simulink subsystem "Controls"  (R2024b)
settings: Solver=VariableStepAuto  StartTime=0.0  StopTime=10.0  RelTol=1e-3
undefined symbols (not defined in the file): D1, DiscIntNeverNeededParam, lag, Tctrl, test_alpha, Ts, Yg
libraries: powerlib_extras x74, simulink x10
(part 1 of 7)
settings Model: ModifiedByFormat=Kyle  Creator=Kyle  LastModifiedBy=Kyle

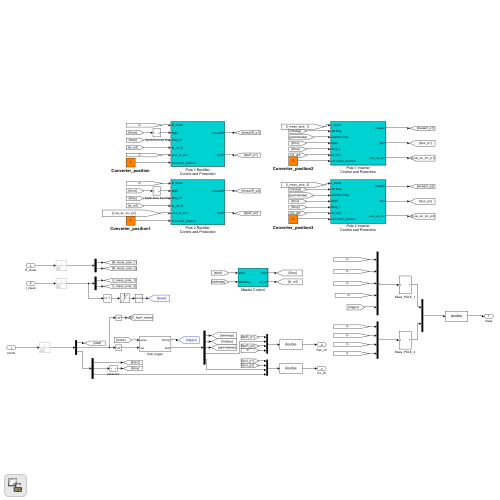
[thumbnail: Simulink's stored preview of the top-level diagram]
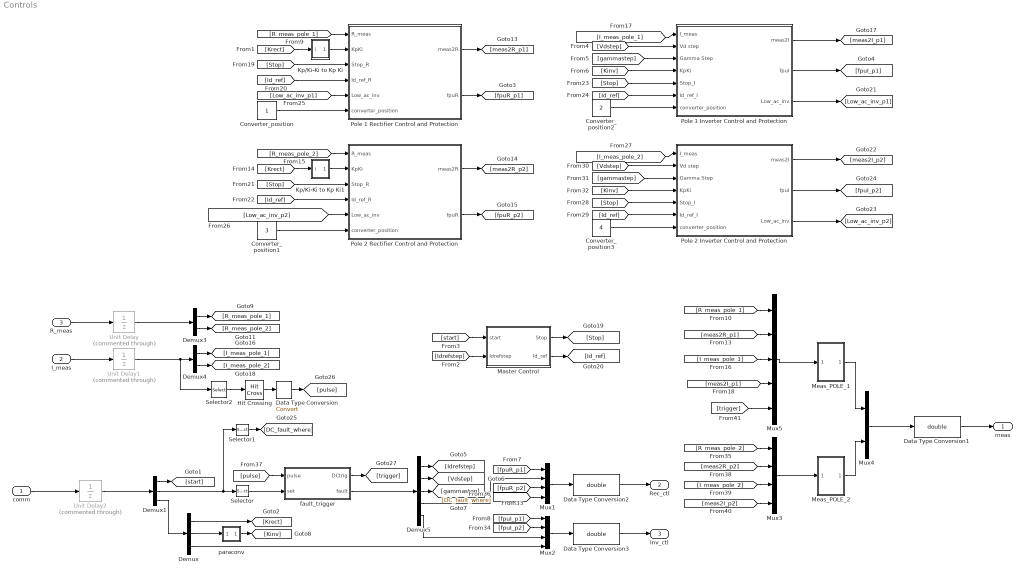
== system Controls ==
  comm : Inport
  I_meas : Inport  Port=2
  R_meas : Inport  Port=3
  Converter_position : Constant
  Converter_position1 : Constant  Value=3
  Converter_position2 : Constant  Value=2
  Converter_position3 : Constant  Value=4
  Data Type Conversion : DataTypeConversion  SaturateOnIntegerOverflow=off  RndMeth=Floor
  Data Type Conversion1 : DataTypeConversion  OutDataTypeStr=double  SaturateOnIntegerOverflow=off  RndMeth=Floor  LockScale=on
  Data Type Conversion2 : DataTypeConversion  OutDataTypeStr=double  SaturateOnIntegerOverflow=off  RndMeth=Floor
  Data Type Conversion3 : DataTypeConversion  OutDataTypeStr=double  SaturateOnIntegerOverflow=off  RndMeth=Floor  LockScale=on
  Demux : Demux  Outputs=[2 6 5]
  Demux1 : Demux  Outputs=[1 16 13]
  Demux3 : Demux  Outputs=[14 14]
  Demux4 : Demux  Outputs=[24 24]
  Demux5 : Demux  Outputs=[1 1 1 2 3]
  Hit Crossing : HitCross  HitCrossingDirection=rising
  Kp/Ki-Ki to Kp Ki : Subsystem
  Kp/Ki-Ki to Kp Ki1 : Subsystem
  Master Control : Subsystem
  Meas_POLE_1 : Subsystem
  Meas_POLE_2 : Subsystem
  Mux1 : Mux  Inputs=[6 2 6 1]
  Mux2 : Mux  Inputs=[6 6 3 5]
  Mux3 : Mux  Inputs=[14 6 24 12 ]
  Mux4 : Mux  Inputs=[57 56]
  Mux5 : Mux  Inputs=[14 6 24 12 1]
  Pole 1 Inverter Control and Protection : Subsystem
  Pole 1 Rectifier Control and Protection : Subsystem
  Pole 2 Inverter Control and Protection : Subsystem
  Pole 2 Rectifier Control and Protection : Subsystem
  Selector : Selector  IndexOptions=Index vector (dialog)  Indices=[1:4, 6:16]  OutputSizes=1
  Selector1 : Selector  IndexOptions=Index vector (dialog)  Indices=[5]  OutputSizes=1
  Selector2 : Selector  IndexOptions=Index vector (dialog)  Indices=1  OutputSizes=1
  Unit Delay : UnitDelay  Commented=through  SampleTime=Ts  HasFrameUpgradeWarning=on
  Unit Delay1 : UnitDelay  Commented=through  SampleTime=Ts  HasFrameUpgradeWarning=on
  Unit Delay2 : UnitDelay  Commented=through  SampleTime=Ts  HasFrameUpgradeWarning=on
  fault_trigger : Subsystem
  paraconv : Subsystem
  meas : Outport
  Rec_ctl : Outport  Port=2
  Inv_ctl : Outport  Port=3
  wires:
  Demux1/1 -> [start]
  [start] -> Master Control/1(start)
  [Idrefstep] -> Master Control/2(Idrefstep)
  [Vdstep] -> Pole 1 Inverter Control and Protection/2(Vd step)
  [gammastep] -> Pole 1 Inverter Control and Protection/3(Gamma Step)
  Pole 1 Inverter Control and Protection/2(fpuI) -> [fpuI_p1]
  Pole 1 Rectifier Control and Protection/2(fpuR) -> [fpuR_p1]
  [Kinv] -> Pole 1 Inverter Control and Protection/4(KpKi)
  Kp/Ki-Ki to Kp Ki/1(o) -> Pole 1 Rectifier Control and Protection/2(KpKi)
  Demux/3 -> Mux2/4
  Demux1/3 -> Demux/1
  [Krect] -> Kp/Ki-Ki to Kp Ki/1(i)
  Demux/1 -> [Krect]
  Demux/2 -> paraconv/1(In1)
  comm/1 -> Unit Delay2/1
  Demux5/1 -> [Idrefstep]
  Demux5/2 -> [Vdstep]
  Demux5/3 -> [gammastep]
  Demux1/2 -> Selector1/1, Selector/1
  paraconv/1(Out1) -> [Kinv]
  [fpuR_p1] -> Mux1/1
  [fpuI_p1] -> Mux2/1
  Demux5/5 -> Mux2/3
  R_meas/1 -> Unit Delay/1
  I_meas/1 -> Unit Delay1/1
  Mux5/1 -> Meas_POLE_1/1(In1)
  Demux3/1 -> [R_meas_pole_1]
  Demux3/2 -> [R_meas_pole_2]
  [R_meas_pole_1] -> Mux5/1
  [R_meas_pole_1] -> Pole 1 Rectifier Control and Protection/1(R_meas)
  Pole 1 Rectifier Control and Protection/1(meas2R) -> [meas2R_p1]
  [meas2R_p1] -> Mux5/2
  Converter_position/1 -> Pole 1 Rectifier Control and Protection/6(converter_position)
  Pole 2 Rectifier Control and Protection/2(fpuR) -> [fpuR_p2]
  Kp/Ki-Ki to Kp Ki1/1(o) -> Pole 2 Rectifier Control and Protection/2(KpKi)
  [Krect] -> Kp/Ki-Ki to Kp Ki1/1(i)
  [R_meas_pole_2] -> Pole 2 Rectifier Control and Protection/1(R_meas)
  Pole 2 Rectifier Control and Protection/1(meas2R) -> [meas2R_p2]
  Converter_position1/1 -> Pole 2 Rectifier Control and Protection/6(converter_position)
  Demux4/1 -> [I_meas_pole_1]
  [I_meas_pole_1] -> Mux5/3
  [I_meas_pole_1] -> Pole 1 Inverter Control and Protection/1(I_meas)
  Pole 1 Inverter Control and Protection/1(meas2I) -> [meas2I_p1]
  [meas2I_p1] -> Mux5/4
  Demux4/2 -> [I_meas_pole_2]
  Converter_position2/1 -> Pole 1 Inverter Control and Protection/7(converter_position)
  Master Control/2(Id_ref) -> [Id_ref]
  Master Control/1(Stop) -> [Stop]
  Pole 1 Inverter Control and Protection/3(Low_ac_inv) -> [Low_ac_inv_p1]
  [Low_ac_inv_p1] -> Pole 1 Rectifier Control and Protection/5(Low_ac_inv)
  [Low_ac_inv_p2] -> Pole 2 Rectifier Control and Protection/5(Low_ac_inv)
  [Vdstep] -> Pole 2 Inverter Control and Protection/2(Vd step)
  [gammastep] -> Pole 2 Inverter Control and Protection/3(Gamma Step)
  Pole 2 Inverter Control and Protection/2(fpuI) -> [fpuI_p2]
  [Kinv] -> Pole 2 Inverter Control and Protection/4(KpKi)
  [I_meas_pole_2] -> Pole 2 Inverter Control and Protection/1(I_meas)
  Pole 2 Inverter Control and Protection/1(meas2I) -> [meas2I_p2]
  Converter_position3/1 -> Pole 2 Inverter Control and Protection/7(converter_position)
  Pole 2 Inverter Control and Protection/3(Low_ac_inv) -> [Low_ac_inv_p2]
  [fpuI_p2] -> Mux2/2
  Mux3/1 -> Meas_POLE_2/1(In1)
  [R_meas_pole_2] -> Mux3/1
  [meas2R_p2] -> Mux3/2
  [I_meas_pole_2] -> Mux3/3
  [meas2I_p2] -> Mux3/4
  Meas_POLE_1/1(Out1) -> Mux4/1
  Meas_POLE_2/1(Out1) -> Mux4/2
  Mux4/1 -> Data Type Conversion1/1
  [Stop] -> Pole 2 Rectifier Control and Protection/3(Stop_R)
  [Id_ref] -> Pole 2 Rectifier Control and Protection/4(Id_ref_R)
  [Id_ref] -> Pole 1 Inverter Control and Protection/6(Id_ref_I)
  [Stop] -> Pole 1 Inverter Control and Protection/5(Stop_I)
  [Stop] -> Pole 2 Inverter Control and Protection/5(Stop_I)
  [Id_ref] -> Pole 2 Inverter Control and Protection/6(Id_ref_I)
  [fpuR_p2] -> Mux1/3
  Demux5/4 -> Mux1/2
  [Stop] -> Pole 1 Rectifier Control and Protection/3(Stop_R)
  [Id_ref] -> Pole 1 Rectifier Control and Protection/4(Id_ref_R)
  Selector/1 -> fault_trigger/2(set)
  [DC_fault_where] -> Mux1/4
  Selector1/1 -> [DC_fault_where]
  fault_trigger/2(fault) -> Demux5/1
  fault_trigger/1(DCtrig) -> [trigger]
  [pulse] -> fault_trigger/1(pulse)
  [trigger] -> Mux5/5
  Hit Crossing/1 -> Data Type Conversion/1
  Data Type Conversion/1 -> [pulse]
  Selector2/1 -> Hit Crossing/1
  Unit Delay/1 -> Demux3/1
  Unit Delay1/1 -> Demux4/1, Selector2/1
  Unit Delay2/1 -> Demux1/1
  Data Type Conversion1/1 -> meas/1
  Mux2/1 -> Data Type Conversion3/1
  Mux1/1 -> Data Type Conversion2/1
  Data Type Conversion2/1 -> Rec_ctl/1
  Data Type Conversion3/1 -> Inv_ctl/1

== system Controls/Kp//Ki-Ki to Kp Ki ==
  i : Inport
  Mux3 : Mux  Inputs=2
  Product11 : Product  Inputs=1  RndMeth=Zero
  Selector12 : Selector  InputPortWidth=2  IndexOptions=Index vector (dialog)  Indices=2  OutputSizes=1
  o : Outport
  wires:
  Mux3/1 -> o/1
  Selector12/1 -> Mux3/2
  Product11/1 -> Mux3/1
  i/1 -> Product11/1, Selector12/1

== system Controls/Kp//Ki-Ki to Kp Ki1 ==
  i : Inport
  Mux3 : Mux  Inputs=2
  Product11 : Product  Inputs=1  RndMeth=Zero
  Selector12 : Selector  InputPortWidth=2  IndexOptions=Index vector (dialog)  Indices=2  OutputSizes=1
  o : Outport
  wires:
  Mux3/1 -> o/1
  Selector12/1 -> Mux3/2
  Product11/1 -> Mux3/1
  i/1 -> Product11/1, Selector12/1

== system Controls/Master Control ==
  note: Master Control
  start : Inport
  Idrefstep : Inport  Port=2
  Constant : Constant  Value=0
  Discrete Monostable1 : powerlib_extras/Discrete  Control Blocks/Discrete Monostable  EdgeDetect=Rising  t_mono=0.1  ic=0  Ts=Tctrl
  Informations : Subsystem
      mask Display: disp('?')
  Product : Product  RndMeth=Zero
  Start/Stop : Subsystem  mask(Start/Stop  & Ramping){Min_ref=0.1, X_start=[0.3333, 0.02], X_up=[5.0, 0.4, 1.0], X_down=[-5.0,  1.4], T_stop=1.6, dt=Tctrl}
      mask prompts: Min_ref "Minimum Steady-State Current Reference (pu):"; X_start "{Start Ramp}: [Rate (pu/s), Time (s)]"; X_up "{Up Ramp}: [Rate (pu/s), Time (s), Final Value (pu)]"; X_down "{Down Ramp}: [Rate (-pu/s), Time (s)]"; T_stop "Stop Time (s):"; dt "Sample Time (s):"
      mask help:
      | At start-up, both converters are deblocked and ramped up to the minimum current (Minimum Steady-State Current Reference) with an adjustable rate (Start Ramp Rate) and application time (Start Ramp Time).
      |
      | After the system stabilisation the current is ramped up to its final value (Up Ramp Final Value) with an adjustable rate (Up Ramp Rate) and execution time (Up Ramp Time).
      |
      | Before stopping the converters (at Stop Time) the current is ramped down to the minimum current  with an adjustable rate (Down Ramp Rate) and execution time  (Down Ramp Time).
      |
      | At Stop Time the reference is ramped down to zero with the same rate used for the Start Ramp.
      mask init:
      | T_up = X_up(2); F_up = X_up(3); up_slope = X_up(1);
      | T_up_final =  T_up + (F_up - Min_ref)/up_slope;
      | 
      | T_down = X_down(2); F_down = Min_ref; down_slope = X_down(1);
      | T_down_final =   T_down + (F_down-F_up)/down_slope;
      | 
      | SS_ramp = X_start(1); T_start = X_start(2);
      | 
      | T_ramp  = [0, T_up, T_up_final,  T_down,  T_down_final, 9999]';
      | U_ramp = [0, 0, F_up-Min_ref,  F_up-Min_ref,  F_down- Min_ref,  F_down - Min_ref]';
      mask Display: disp('Start/Stop\n & Ramping')
  Step : Step  Time=0.1  SampleTime=Tctrl
  Sum : Sum  SaturateOnIntegerOverflow=on
  Sum1 : Sum  SaturateOnIntegerOverflow=on
  g : Gain  Gain=-0.2  SaturateOnIntegerOverflow=on  OutDataTypeStr=Inherit: Same as input  ParamDataTypeStr=Inherit: Same as input
  Stop : Outport
  Id_ref : Outport  Port=2
  wires:
  Start/Stop/2("Stop ") -> Stop/1
  Step/1 -> Product/1
  Product/1 -> Start/Stop/1(start)
  start/1 -> Product/2
  Idrefstep/1 -> Discrete Monostable1/1
  g/1 -> Sum1/2
  Discrete Monostable1/1 -> g/1
  Start/Stop/1(Id_ref_ramp) -> Sum/1
  Sum/1 -> Id_ref/1
  Sum1/1 -> Sum/2
  Constant/1 -> Sum1/1

== system Controls/Meas_POLE_1 ==
  In1 : Inport
  Demux1 : Demux  Outputs="[14 6 24 12  1]"
      settings: DisplayOption=none
  Demux3 : Demux  Outputs=12
      settings: DisplayOption=none
  Demux4 : Demux  Outputs=14
      settings: DisplayOption=none
  Demux5 : Demux  Outputs=6
      settings: DisplayOption=none
  Demux6 : Demux  Outputs=24
      settings: DisplayOption=none
  Mux1 : Mux  Inputs="[14 6 24 12  1]"
  Mux3 : Mux  Inputs=12
  Mux4 : Mux  Inputs=14
  Mux5 : Mux  Inputs=24
  Mux6 : Mux  Inputs=6
  Out1 : Outport
  wires:
  Demux6/24 -> Mux5/24  "Iac fault (A)"
  Demux4/14 -> Mux4/14  "Idc fault (A)"
  Demux1/2 -> Demux5/1
  Mux6/1 -> Mux1/2
  Demux5/1 -> Mux6/1  "Vdc_Rect (pu/500kV)"
  Demux5/2 -> Mux6/2  "Id_ref_limit_Rect"
  Demux5/3 -> Mux6/3  "alpha Rect (degree)"
  Demux5/4 -> Mux6/4  "Mode"
  Demux5/5 -> Mux6/5  "Low AC voltage Rect"
  Demux5/6 -> Mux6/6  "Forced alpha Rect"
  Demux1/1 -> Demux4/1
  Demux4/13 -> Mux4/13  "Vdc_neutral (pu/500kV)"
  Demux4/12 -> Mux4/12  "Ithy1 D Rect (pu/1kA)"
  Demux4/11 -> Mux4/11  "Vthy1 D Rect (pu/500kV)"
  Demux4/10 -> Mux4/10  "Ithy1 Y Rect (pu/1kA)"
  Demux4/9 -> Mux4/9  "Vthy1 Y Rect (pu/500kV)"
  Demux4/8 -> Mux4/8  "Id Rect (pu/1kA)"
  Demux4/7 -> Mux4/7  "Vdc Rect (pu/500kV)"
  Mux4/1 -> Mux1/1
  Demux4/6 -> Mux4/6  "Ic Rect (pu/817A)"
  Demux4/5 -> Mux4/5  "Ib Rect (pu/817A)"
  Demux4/4 -> Mux4/4  "Ia Rect (pu/817A)"
  Demux4/3 -> Mux4/3  "Vc_Rect (pu/500kVLL)"
  Demux4/2 -> Mux4/2  "Vb_Rect (pu/500kVLL)"
  Demux4/1 -> Mux4/1  "Va_Rect (pu/500kVLL)"
  Mux3/1 -> Mux1/4
  Demux1/4 -> Demux3/1
  Demux3/12 -> Mux3/12  "Gamma mean"
  Demux3/11 -> Mux3/11  "Vsw1 Inv(pu)"
  Demux3/10 -> Mux3/10  "Isw1 Inv (pu)"
  Demux3/9 -> Mux3/9  "Alpha  min Inv"
  Demux3/8 -> Mux3/8  "Low AC voltage Inv"
  Demux3/7 -> Mux3/7  "Gamma Ref Inv"
  Demux3/6 -> Mux3/6  "Gamma min Inv"
  Demux3/5 -> Mux3/5  "Mode"
  Demux3/4 -> Mux3/4  "alpha Inv (degree)"
  Demux3/3 -> Mux3/3  "Id limite (pu)"
  Demux3/2 -> Mux3/2  "Vd Ref Inv (pu)"
  Demux3/1 -> Mux3/1  "Vdc_Inv (pu/500kV)"
  Demux1/5 -> Mux1/5  "trigger sig"
  In1/1 -> Demux1/1
  Mux1/1 -> Out1/1
  Demux6/23 -> Mux5/23  "Vdc_neutral (pu/500kV)"
  Demux6/22 -> Mux5/22  "V thy 1D (pu/500kV)"
  Demux6/21 -> Mux5/21  "Vthy1Y(pu/500kV)"
  Demux6/20 -> Mux5/20  "I thy 6 D (pu/1kA)"
  Demux6/19 -> Mux5/19  "I thy 5 D (pu/1kA)"
  Demux6/18 -> Mux5/18  "I thy 4 D (pu/1kA)"
  Demux6/17 -> Mux5/17  "I thy 3 D (pu/1kA)"
  Demux6/16 -> Mux5/16  "I thy 2 D (pu/1kA)"
  Demux6/15 -> Mux5/15  "I thy 1 D (pu/1kA)"
  Demux6/14 -> Mux5/14  "I thy 6 Y (pu/1kA)"
  Demux6/1 -> Mux5/1  "Va_Inv (pu/345kVLL)"
  Demux6/2 -> Mux5/2  "Vb_Inv (pu/345kVLL)"
  Demux6/3 -> Mux5/3  "Vc_Inv (pu/345kVLL)"
  Demux6/4 -> Mux5/4  "Ia_Inv (pu/290A)"
  Demux6/5 -> Mux5/5  "Ib_Inv (pu/290A)"
  Demux6/6 -> Mux5/6  "Ic_Inv (pu/290A)"
  Demux1/3 -> Demux6/1
  Mux5/1 -> Mux1/3
  Demux6/7 -> Mux5/7  "Vdc Inv (pu/500kV)"
  Demux6/8 -> Mux5/8  "Idc Inv (pu/1kA)"
  Demux6/9 -> Mux5/9  "I thy 1 Y (pu/1kA)"
  Demux6/10 -> Mux5/10  "I thy 2 Y (pu/1kA)"
  Demux6/11 -> Mux5/11  "I thy 3 Y (pu/1kA)"
  Demux6/12 -> Mux5/12  "I thy 4 Y (pu/1kA)"
  Demux6/13 -> Mux5/13  "I thy 5 Y (pu/1kA)"

== system Controls/Meas_POLE_2 ==
  In1 : Inport
  Demux1 : Demux  Outputs=[14 6 24 12]
      settings: DisplayOption=none
  Demux3 : Demux  Outputs=12
      settings: DisplayOption=none
  Demux4 : Demux  Outputs=14
      settings: DisplayOption=none
  Demux5 : Demux  Outputs=6
      settings: DisplayOption=none
  Demux6 : Demux  Outputs=24
      settings: DisplayOption=none
  Gain{,1..4} (5 alike) : Gain  Gain=-1
  Mux1 : Mux  Inputs=[14 6 24 12 ]
  Mux3 : Mux  Inputs=12
  Mux4 : Mux  Inputs=14
  Mux5 : Mux  Inputs=24
  Mux6 : Mux  Inputs=6
  Out1 : Outport
  wires:
  Gain4/1 -> Mux3/3  "Id limite (pu)"
  Gain3/1 -> Mux3/2  "Vd Ref Inv (pu)"
  Gain2/1 -> Mux3/1  "Vdc_Inv (pu/500kV)"
  Gain1/1 -> Mux6/2  "Id_ref_limit_Rect"
  Gain/1 -> Mux6/1  "Vdc_Rect (pu/500kV)"
  Demux6/24 -> Mux5/24  "Iac fault (A)"
  Demux4/14 -> Mux4/14  "Idc fault (A)"
  Demux1/2 -> Demux5/1
  Mux6/1 -> Mux1/2
  Demux5/1 -> Gain/1
  Demux5/2 -> Gain1/1
  Demux5/3 -> Mux6/3  "alpha Rect (degree)"
  Demux5/4 -> Mux6/4  "Mode"
  Demux5/5 -> Mux6/5  "Low AC voltage Rect"
  Demux5/6 -> Mux6/6  "Forced alpha Rect"
  Demux1/1 -> Demux4/1
  Demux4/13 -> Mux4/13  "Vdc_neutral (pu/500kV)"
  Demux4/12 -> Mux4/12  "Ithy1 D Rect (pu/1kA)"
  Demux4/11 -> Mux4/11  "Vthy1 D Rect (pu/500kV)"
  Demux4/10 -> Mux4/10  "Ithy1 Y Rect (pu/1kA)"
  Demux4/9 -> Mux4/9  "Vthy1 Y Rect (pu/500kV)"
  Demux4/8 -> Mux4/8  "Id Rect (pu/1kA)"
  Demux4/7 -> Mux4/7  "Vdc Rect (pu/500kV)"
  Mux4/1 -> Mux1/1
  Demux4/6 -> Mux4/6  "Ic Rect (pu/817A)"
  Demux4/5 -> Mux4/5  "Ib Rect (pu/817A)"
  Demux4/4 -> Mux4/4  "Ia Rect (pu/817A)"
  Demux4/3 -> Mux4/3  "Vc_Rect (pu/500kVLL)"
  Demux4/2 -> Mux4/2  "Vb_Rect (pu/500kVLL)"
  Demux4/1 -> Mux4/1  "Va_Rect (pu/500kVLL)"
  Mux3/1 -> Mux1/4
  Demux1/4 -> Demux3/1
  Demux3/12 -> Mux3/12  "Gamma mean"
  Demux3/11 -> Mux3/11  "Vsw1 Inv(pu)"
  Demux3/10 -> Mux3/10  "Isw1 Inv (pu)"
  Demux3/9 -> Mux3/9  "Alpha  min Inv"
  Demux3/8 -> Mux3/8  "Low AC voltage Inv"
  Demux3/7 -> Mux3/7  "Gamma Ref Inv"
  Demux3/6 -> Mux3/6  "Gamma min Inv"
  Demux3/5 -> Mux3/5  "Mode"
  Demux3/4 -> Mux3/4  "alpha Inv (degree)"
  Demux3/3 -> Gain4/1
  Demux3/2 -> Gain3/1
  Demux3/1 -> Gain2/1
  In1/1 -> Demux1/1
  Mux1/1 -> Out1/1
  Demux6/23 -> Mux5/23  "Vdc_neutral (pu/500kV)"
  Demux6/22 -> Mux5/22  "V thy 1D (pu/500kV)"
  Demux6/21 -> Mux5/21  "Vthy1Y(pu/500kV)"
  Demux6/20 -> Mux5/20  "I thy 6 D (pu/1kA)"
  Demux6/19 -> Mux5/19  "I thy 5 D (pu/1kA)"
  Demux6/18 -> Mux5/18  "I thy 4 D (pu/1kA)"
  Demux6/17 -> Mux5/17  "I thy 3 D (pu/1kA)"
  Demux6/16 -> Mux5/16  "I thy 2 D (pu/1kA)"
  Demux6/15 -> Mux5/15  "I thy 1 D (pu/1kA)"
  Demux6/14 -> Mux5/14  "I thy 6 Y (pu/1kA)"
  Demux6/1 -> Mux5/1  "Va_Inv (pu/345kVLL)"
  Demux6/2 -> Mux5/2  "Vb_Inv (pu/345kVLL)"
  Demux6/3 -> Mux5/3  "Vc_Inv (pu/345kVLL)"
  Demux6/4 -> Mux5/4  "Ia_Inv (pu/1183A)"
  Demux6/5 -> Mux5/5  "Ib_Inv (pu/1183A)"
  Demux6/6 -> Mux5/6  "Ic_Inv (pu/1183A)"
  Demux1/3 -> Demux6/1
  Mux5/1 -> Mux1/3
  Demux6/7 -> Mux5/7  "Vdc Inv (pu/500kV)"
  Demux6/8 -> Mux5/8  "Idc Inv (pu/1kA)"
  Demux6/9 -> Mux5/9  "I thy 1 Y (pu/1kA)"
  Demux6/10 -> Mux5/10  "I thy 2 Y (pu/1kA)"
  Demux6/11 -> Mux5/11  "I thy 3 Y (pu/1kA)"
  Demux6/12 -> Mux5/12  "I thy 4 Y (pu/1kA)"
  Demux6/13 -> Mux5/13  "I thy 5 Y (pu/1kA)"

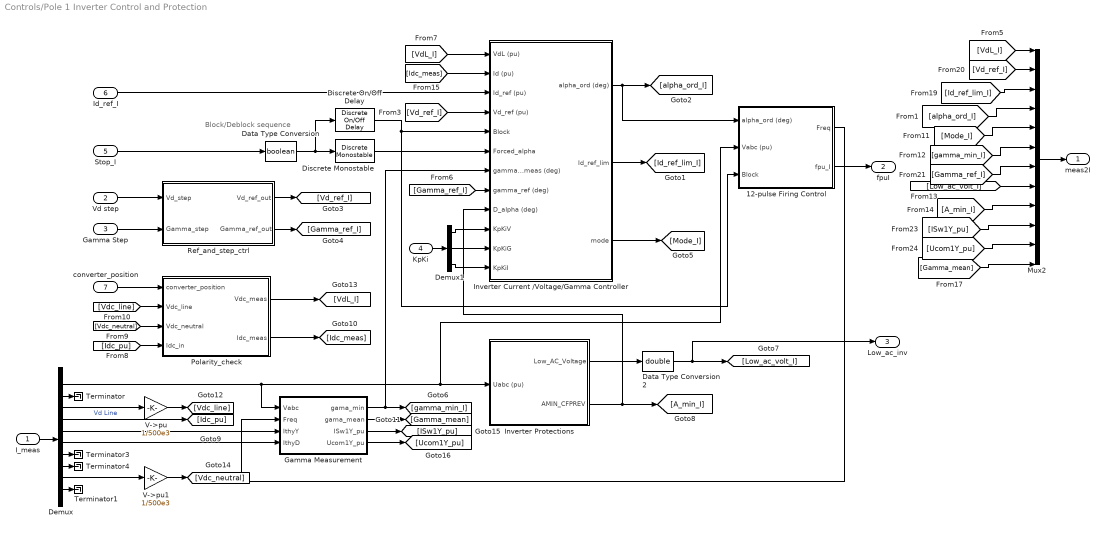
== system Controls/Pole 1 Inverter Control and Protection ==
  note: Block/Deblock sequence
  I_meas : Inport
  Vd step : Inport  Port=2
  Gamma Step : Inport  Port=3
  KpKi : Inport  Port=4
  Stop_I : Inport  Port=5
  Id_ref_I : Inport  Port=6
  converter_position : Inport  Port=7
  12-pulse Firing Control : Subsystem  mask(HVDC Discrete 12-pulse Firing Control){Pw=101.5, PLL_PF=[0,  50], PLL_G=[60, 1400], dt=Tctrl}
      mask prompts: Pw "{Pulse Generator}: Pulse Width (deg)"; PLL_PF "{PLL}: Initial [Phase (deg) Frequency (Hz)]"; PLL_G "{PLL}: Regulator gains [Kp (rad)  Ki (rad/s)]"; dt "Sample Time (s):"
      mask help:
      | This block contains a PLL and a 12-pulse generator to provide the firing pulses to the HVDC converter.
      | The firing control is of the equidistant type. It is based on a Phase Locked Loop (PLL) synchronized on positive-sequence of the fundamental voltage.
      mask init:
      | PLL_ph = PLL_PF(1); PLL_f0 = PLL_PF(2);
      | PLL_Kp = PLL_G(1); PLL_Ki = PLL_G(2);
      mask Help:
      | INPUTS:
      | alpha :  Desired firing angle of thyristors (deg).
      | Vabc  : 3 phase-to-ground voltages (pu)  on the primary winding of the YgYD converter transformer
      | Block  : Logical signal  (0-1). The pulses are not generated when the value is 1.
      | 
      | 
      | 
      | OUTPUTS:
      |  PulsesY :  6 pulses to be sent to the half converter connected to the Wye winding.
      |  PulsesD :  6 pulses to be sent to the half converter connected to the Delta winding.
  Data Type Conversion : DataTypeConversion  OutDataTypeStr=boolean
  Data Type Conversion2 : DataTypeConversion  OutDataTypeStr=double
  Demux : Demux  Outputs="[3 3 1 1 6 6 1  1 1 1]"
  Demux1 : Demux  Outputs=[2 2 2]
  Discrete Monostable : powerlib_extras/Discrete  Control Blocks/Discrete Monostable  EdgeDetect=Rising  t_mono=0.15  ic=1  Ts=Tctrl
  Discrete On/Off Delay : powerlib_extras/Discrete  Control Blocks/Discrete On//Off Delay  type_delay=On delay  delay=0.1  ic=1  Ts=Tctrl
  Gamma Measurement : Subsystem
  "Inverter Current /Voltage/Gamma Controller " : Subsystem  mask(Discrete HVDC Controller){Mode=Inverter (Current + Voltage + Gamma), XPILim=[166, 92], XLin=[160, 120], XKPI_I=[45, 4500, 90], Id_marg=0.1, XKPI_V=[35, 2250,  90], Vd_marg=0.05, XKPI_G=[1, 20,  90 ], G_marg=1, T_I=0.3e-3, XT_V=[15,  0.707], Xvdcol=[0.6, 0.18, 0.30, 0.1, 0.080], alpha_const=off, Xalpha_fix=[92, inf, -1000], dt=Tctrl}
      mask prompts: Mode "Control Mode :"; XPILim "{Alpha Limits}  [alpha max (deg), alpha min (deg) ]"; XLin "Kp Lin. Angle Limits (alpha or beta) : [Max  (deg), Min  (deg) ]"; XKPI_I "{Current Regulator}   [Kp (deg/pu) , Ki (deg/pu/s), AlphaInit (deg) ]"; Id_marg "Current Margin (pu) :"; XKPI_V "{Voltage Regulator}   [Kp (deg/pu) , Ki (deg/pu/s),  AlphaInit (deg) ]"; Vd_marg "Voltage Margin (pu):"; XKPI_G "{Gamma Regulator} [Kp, Ki (s), AlphaInit (deg)]"; G_marg "Gamma Margin (deg):"; T_I "{Id Meas. Filter H(s)=1/(1+Ts)} T(s):"; XT_V "{Vd Meas. Low-Pass 2nd Order Filter}  [fo,  Zeta ]"; Xvdcol "{VDCOL}  [ VdThresh.(pu),VdMin(pu),IdMin(pu),IdMinAbs(pu),Tup(s) ]"; alpha_const "Constant alpha mode"; Xalpha_fix "{Ct.  or Forced alpha)}  [Alpha (deg), + Rate limit, - Rate limit (deg/s)]"; dt "Sample Time (s):"
      mask help:
      | This block contains the regulators and functions to control the firing angle alpha of a HVDC rectifier or inverter.
      |  See the 'HVDC Transmission System' case study of the User's Manual for description of the block functionality.
      mask init:
      | % Max_lin = max(180-Xlin)  Min_lin = min(180-Xlin)
      | 
      | alpha_max = XPILim(1); alpha_min = XPILim(2);
      | alpha_fix = Xalpha_fix(1); PRate_fix = Xalpha_fix(2);NRate_fix = Xalpha_fix(3);
      | Kp_I = XKPI_I(1); Ki_I = XKPI_I(2); ICi_I = XKPI_I(3);
      | Kp_V = XKPI_V(1); Ki_V = XKPI_V(2); ICi_V = XKPI_V(3);
      | Kp_G = XKPI_G(1); Ki_G = XKPI_G(2); ICi_G = XKPI_G(3);
      | f0_V = XT_V(1); Z_V = XT_V(2);
      | 
      | Inverter = Mode > 1;
      | 
      | if (Mode == 1) 
      | 	Id_marg = 0.0;
      | 	Max_lin = 60; Min_lin = 20;
      | else
      | 	Max_lin = 160; Min_lin = 120;
      | end;
      | 
      | 
      | Vd_seuil = Xvdcol(1); Vd_min=Xvdcol(2);Id_min=Xvdcol(3);Id_min_abs=Xvdcol(4);Tup=Xvdcol(5);
      | if strcmp(alpha_const,'on'), test_alpha = true; else, test_alpha = false; end
      mask TypeOptions Mode: Rectifier (Current) | Inverter (Current + Voltage + Gamma) | Inverter (Current + Voltage) | Inverter (Current + Gamma)
      mask Callback Mode:
      | mode=get_param(gcb,'Mode');
      | 
      | cb=get_param(gcb,'MaskVisibilities');
      | 
      | if strcmp(mode,'Rectifier (Current)')
      | 	cb{10}='on';
      |     cb{11} = 'off';
      | 
      | 	 cb{3}='off';
      | 	 cb{5}='off';cb{6}='off';cb{7}='off';cb{8}='off';cb{9}='off';
      |     set_param(gcb,'MaskVisibilities',cb);
      | elseif (strcmp(mode,'Inverter (Current + Voltage + Gamma)'))
      | 	 cb{3}='off';
      | 	 cb{5}='on';cb{6}='on';cb{7}='on';cb{8}='on';cb{9}='on';cb{11} = 'on';
      | 	 set_param(gcb,'MaskVisibilities',cb);
      | elseif (strcmp(mode,'Inverter (Current + Voltage)'))
      | 	 cb{3}='off';
      | 	 cb{5}='on';cb{6}='on';cb{7}='on';cb{8}='off';cb{9}='off'; cb{11} = 'on';
      |      set_param(gcb,'MaskVisibilities',cb);
      | else
      | 	 cb{3}='off';
      | 	 cb{5}='on';cb{6}='off';cb{7}='off';cb{8}='on';cb{9}='on'; cb{11} = 'on';
      | 	 set_param(gcb,'MaskVisibilities',cb);
      | end
  Inverter Protections : Subsystem  TreatAsAtomicUnit=on  mask(Protection LACVD a Radisson (cyc = 1 ms)){}
  Mux2 : Mux  Inputs=12
  Polarity_check : Subsystem
  Ref_and_step_ctrl : Subsystem
  Terminator{,1,3..4} (4 alike) : Terminator
  V->pu : Gain  Gain=1/500e3  SaturateOnIntegerOverflow=on  OutDataTypeStr=Inherit: Same as input  ParamDataTypeStr=Inherit: Same as input
  V->pu1 : Gain  Gain=1/500e3  SaturateOnIntegerOverflow=on  OutDataTypeStr=Inherit: Same as input  ParamDataTypeStr=Inherit: Same as input
  meas2I : Outport
  fpuI : Outport  Port=2
  Low_ac_inv : Outport  Port=3
  wires:
  V->pu1/1 -> [Vdc_neutral]
  Gamma Measurement/4(Ucom1Y_pu) -> [Ucom1Y_pu]
  Gamma Measurement/3(ISw1Y_pu) -> [ISw1Y_pu]
  Demux/1 -> 12-pulse Firing Control/2(Vabc (pu)), Inverter Protections/1(Uabc (pu)), Gamma Measurement/1(Vabc)
  [Idc_meas] -> "Inverter Current /Voltage/Gamma Controller "/2(Id (pu))
  Demux/9 -> V->pu1/1
  Demux/10 -> Terminator1/1
  Polarity_check/2(Idc_meas) -> [Idc_meas]
  [Vdc_neutral] -> Polarity_check/3(Vdc_neutral)
  [Vdc_line] -> Polarity_check/2(Vdc_line)
  converter_position/1 -> Polarity_check/1(converter_position)
  Polarity_check/1(Vdc_meas) -> [VdL_I]
  [Idc_pu] -> Polarity_check/4(Idc_in)
  Gamma Step/1 -> Ref_and_step_ctrl/2(Gamma_step)
  Ref_and_step_ctrl/2(Gamma_ref_out) -> [Gamma_ref_I]
  Vd step/1 -> Ref_and_step_ctrl/1(Vd_step)
  Ref_and_step_ctrl/1(Vd_ref_out) -> [Vd_ref_I]
  Demux1/1 -> "Inverter Current /Voltage/Gamma Controller "/10(KpKiV)
  Demux1/3 -> "Inverter Current /Voltage/Gamma Controller "/12(KpKiI)
  Demux1/2 -> "Inverter Current /Voltage/Gamma Controller "/11(KpKiG)
  KpKi/1 -> Demux1/1
  12-pulse Firing Control/2(fpu_I) -> fpuI/1
  12-pulse Firing Control/1(Freq) -> Gamma Measurement/2(Freq)
  Data Type Conversion2/1 -> Low_ac_inv/1, [Low_ac_volt_I]
  [Gamma_mean] -> Mux2/12
  [Ucom1Y_pu] -> Mux2/11
  [ISw1Y_pu] -> Mux2/10
  [A_min_I] -> Mux2/9
  [Low_ac_volt_I] -> Mux2/8
  [Gamma_ref_I] -> Mux2/7
  [gamma_min_I] -> Mux2/6
  [Mode_I] -> Mux2/5
  [alpha_ord_I] -> Mux2/4
  [Id_ref_lim_I] -> Mux2/3
  [Vd_ref_I] -> Mux2/2
  [VdL_I] -> Mux2/1
  Mux2/1 -> meas2I/1
  Demux/8 -> Terminator4/1
  Demux/7 -> Terminator3/1
  Demux/6 -> Gamma Measurement/4(IthyD)
  Demux/5 -> Gamma Measurement/3(IthyY)
  Demux/3 -> V->pu/1  "Vd Line"
  Demux/2 -> Terminator/1
  I_meas/1 -> Demux/1
  Discrete Monostable/1 -> "Inverter Current /Voltage/Gamma Controller "/6(Forced_alpha)
  [Vd_ref_I] -> "Inverter Current /Voltage/Gamma Controller "/4(Vd_ref (pu))
  Discrete On/Off Delay/1 -> 12-pulse Firing Control/3(Block), "Inverter Current /Voltage/Gamma Controller "/5(Block)
  Id_ref_I/1 -> "Inverter Current /Voltage/Gamma Controller "/3(Id_ref (pu))
  Demux/4 -> [Idc_pu]
  [VdL_I] -> "Inverter Current /Voltage/Gamma Controller "/1(VdL (pu))
  "Inverter Current /Voltage/Gamma Controller "/3(mode) -> [Mode_I]
  "Inverter Current /Voltage/Gamma Controller "/2(Id_ref_lim) -> [Id_ref_lim_I]
  "Inverter Current /Voltage/Gamma Controller "/1(alpha_ord (deg)) -> 12-pulse Firing Control/1(alpha_ord (deg)), [alpha_ord_I]
  Gamma Measurement/2(gama_mean) -> [Gamma_mean]
  Gamma Measurement/1(gama_min) -> [gamma_min_I], "Inverter Current /Voltage/Gamma Controller "/7(gamma_meas (deg))
  [Gamma_ref_I] -> "Inverter Current /Voltage/Gamma Controller "/8(gamma_ref (deg))
  V->pu/1 -> [Vdc_line]
  Inverter Protections/1(Low_AC_Voltage) -> Data Type Conversion2/1
  Inverter Protections/2(AMIN_CFPREV) -> "Inverter Current /Voltage/Gamma Controller "/9(D_alpha (deg)), [A_min_I]
  Stop_I/1 -> Data Type Conversion/1
  Data Type Conversion/1 -> Discrete Monostable/1, Discrete On/Off Delay/1

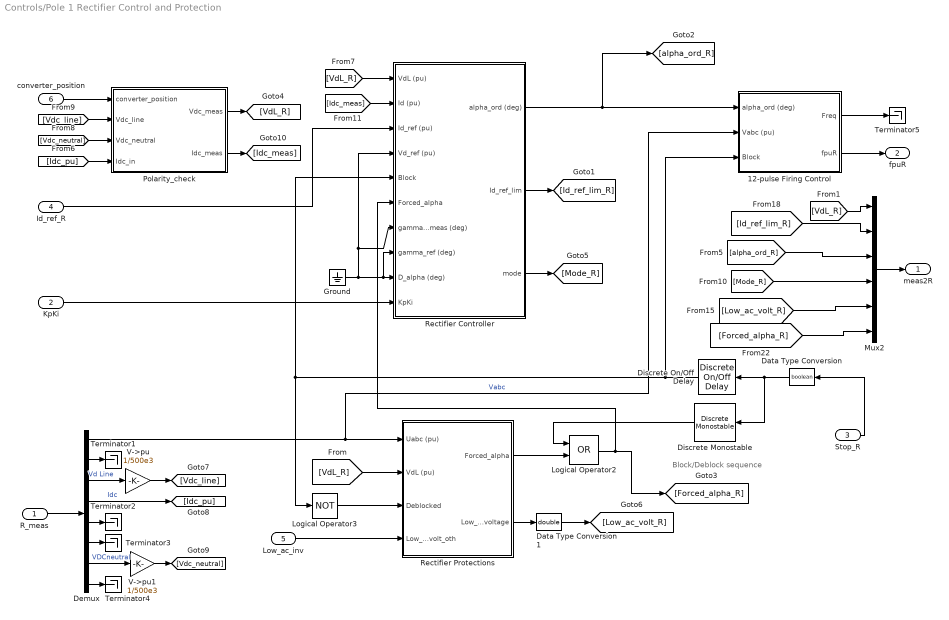
== system Controls/Pole 1 Rectifier Control and Protection ==
  note: Block/Deblock sequence
  R_meas : Inport
  KpKi : Inport  Port=2
  Stop_R : Inport  Port=3
  Id_ref_R : Inport  Port=4
  Low_ac_inv : Inport  Port=5
  converter_position : Inport  Port=6
  12-pulse Firing Control : Subsystem  mask(HVDC Discrete 12-pulse Firing Control){Pw=101.5, PLL_PF=[0,  60], PLL_G=[60, 1400], dt=Tctrl}
      mask prompts: Pw "{Pulse Generator}: Pulse Width (deg)"; PLL_PF "{PLL}: Initial [Phase (deg) Frequency (Hz)]"; PLL_G "{PLL}: Regulator gains [Kp (rad)  Ki (rad/s)]"; dt "Sample Time (s):"
      mask help:
      | This block contains a PLL and a 12-pulse generator to provide the firing pulses to the HVDC converter.
      | The firing control is of the equidistant type. It is based on a Phase Locked Loop (PLL) synchronized on positive-sequence of the fundamental voltage.
      mask init:
      | PLL_ph = PLL_PF(1); PLL_f0 = PLL_PF(2);
      | PLL_Kp = PLL_G(1); PLL_Ki = PLL_G(2);
      mask Help:
      | INPUTS:
      | alpha :  Desired firing angle of thyristors (deg).
      | Vabc  : 3 phase-to-ground voltages (pu)  on the primary winding of the YgYD converter transformer
      | Block  : Logical signal  (0-1). The pulses are not generated when the value is 1.
      | 
      | 
      | 
      | OUTPUTS:
      |  PulsesY :  6 pulses to be sent to the half converter connected to the Wye winding.
      |  PulsesD :  6 pulses to be sent to the half converter connected to the Delta winding.
  Data Type Conversion : DataTypeConversion  OutDataTypeStr=boolean
  Data Type Conversion1 : DataTypeConversion  OutDataTypeStr=double
  Demux : Demux  Outputs=[3 3 1 1 2 2 1 1]
  Discrete Monostable : powerlib_extras/Discrete  Control Blocks/Discrete Monostable  EdgeDetect=Rising  t_mono=0.15  ic=1  Ts=Tctrl
  Discrete On/Off Delay : powerlib_extras/Discrete  Control Blocks/Discrete On//Off Delay  type_delay=On delay  delay=0.1  ic=1  Ts=Tctrl
  Ground : Ground
  Logical Operator2 : Logic  Operator=OR  AllPortsSameDT=off
  Logical Operator3 : Logic  Operator=NOT
  Mux2 : Mux  Inputs=6
  Polarity_check : Subsystem
  Rectifier Controller : Subsystem  mask(Discrete HVDC Controller){Mode=Rectifier (Current), XPILim=[166, 5], XLin=[160, 120], XKPI_I=[45, 4500, 90], Id_marg=0.1, XKPI_V=[35, 2250,  90], Vd_marg=0.05, XKPI_G=[1, 20,  90 ], G_marg=1, T_I=0.3e-3, XT_V=[15,  0.707], Xvdcol=[0.6, 0.18, 0.30, 0.1, 0.080], alpha_const=off, Xalpha_fix=[166, inf, -inf], dt=Tctrl}
      mask prompts: Mode "Control Mode :"; XPILim "{Alpha Limits}  [alpha max (deg), alpha min (deg) ]"; XLin "Kp Lin. Angle Limits (alpha or beta) : [Max  (deg), Min  (deg) ]"; XKPI_I "{Current Regulator}   [Kp (deg/pu) , Ki (deg/pu/s), AlphaInit (deg) ]"; Id_marg "Current Margin (pu) :"; XKPI_V "{Voltage Regulator}   [Kp (deg/pu) , Ki (deg/pu/s),  AlphaInit (deg) ]"; Vd_marg "Voltage Margin (pu):"; XKPI_G "{Gamma Regulator} [Kp, Ki (s), AlphaInit (deg)]"; G_marg "Gamma Margin (deg):"; T_I "{Id Meas. Filter H(s)=1/(1+Ts)} T(s):"; XT_V "{Vd Meas. Low-Pass 2nd Order Filter}  [fo,  Zeta ]"; Xvdcol "{VDCOL}  [ VdThresh.(pu),VdMin(pu),IdMin(pu),IdMinAbs(pu),Tup(s) ]"; alpha_const "Constant alpha mode"; Xalpha_fix "{Ct.  or Forced alpha)}  [Alpha (deg), + Rate limit, - Rate limit (deg/s)]"; dt "Sample Time (s):"
      mask help:
      | This block contains the regulators and functions to control the firing angle alpha of a HVDC rectifier or inverter.
      |  See the 'HVDC Transmission System' case study of the User's Manual for description of the block functionality.
      mask init: same as Controls/Pole 1 Inverter Control and Protection/Inverter Current /Voltage/Gamma Controller 
      mask TypeOptions Mode: Rectifier (Current) | Inverter (Current + Voltage + Gamma) | Inverter (Current + Voltage) | Inverter (Current + Gamma)
      mask Callback Mode:
      | mode=get_param(gcb,'Mode');
      | 
      | cb=get_param(gcb,'MaskVisibilities');
      | 
      | if strcmp(mode,'Rectifier (Current)')
      | 	cb{10}='on';
      |     cb{11} = 'off';
      | 
      | 	 cb{3}='off';
      | 	 cb{5}='off';cb{6}='off';cb{7}='off';cb{8}='off';cb{9}='off';
      |     set_param(gcb,'MaskVisibilities',cb);
      | elseif (strcmp(mode,'Inverter (Current + Voltage + Gamma)'))
      | 	 cb{3}='off';
      | 	 cb{5}='on';cb{6}='on';cb{7}='on';cb{8}='on';cb{9}='on';cb{11} = 'on';
      | 	 set_param(gcb,'MaskVisibilities',cb);
      | elseif (strcmp(mode,'Inverter (Current + Voltage)'))
      | 	 cb{3}='off';
      | 	 cb{5}='on';cb{6}='on';cb{7}='on';cb{8}='off';cb{9}='off'; cb{11} = 'on';
      |      set_param(gcb,'MaskVisibilities',cb);
      | else
      | 	 cb{3}='off';
      | 	 cb{5}='on';cb{6}='off';cb{7}='off';cb{8}='on';cb{9}='on'; cb{11} = 'on';
      | 	 set_param(gcb,'MaskVisibilities',cb);
      | end
  Rectifier Protections : Subsystem  TreatAsAtomicUnit=on  mask(Protection LACVD a Radisson (cyc = 1 ms)){}
  Terminator{1..5} (5 alike) : Terminator
  V->pu : Gain  Gain=1/500e3  SaturateOnIntegerOverflow=on  OutDataTypeStr=Inherit: Same as input  ParamDataTypeStr=Inherit: Same as input
  V->pu1 : Gain  Gain=1/500e3  SaturateOnIntegerOverflow=on  OutDataTypeStr=Inherit: Same as input  ParamDataTypeStr=Inherit: Same as input
  meas2R : Outport
  fpuR : Outport  Port=2
  wires:
  Logical Operator2/1 -> Rectifier Controller/6(Forced_alpha), [Forced_alpha_R]
  V->pu1/1 -> [Vdc_neutral]
  Id_ref_R/1 -> Rectifier Controller/3(Id_ref (pu))
  [Idc_meas] -> Rectifier Controller/2(Id (pu))
  Polarity_check/2(Idc_meas) -> [Idc_meas]
  [Vdc_neutral] -> Polarity_check/3(Vdc_neutral)
  [Vdc_line] -> Polarity_check/2(Vdc_line)
  converter_position/1 -> Polarity_check/1(converter_position)
  Polarity_check/1(Vdc_meas) -> [VdL_R]
  [Idc_pu] -> Polarity_check/4(Idc_in)
  Demux/7 -> V->pu1/1  "VDCneutral"
  Demux/8 -> Terminator4/1
  KpKi/1 -> Rectifier Controller/10(KpKi)
  12-pulse Firing Control/2(fpuR) -> fpuR/1
  12-pulse Firing Control/1(Freq) -> Terminator5/1
  Data Type Conversion1/1 -> [Low_ac_volt_R]
  Mux2/1 -> meas2R/1
  [Forced_alpha_R] -> Mux2/6
  [Low_ac_volt_R] -> Mux2/5
  [Mode_R] -> Mux2/4
  [alpha_ord_R] -> Mux2/3
  [Id_ref_lim_R] -> Mux2/2
  [VdL_R] -> Mux2/1
  Demux/6 -> Terminator3/1
  Demux/5 -> Terminator2/1
  Demux/2 -> Terminator1/1
  R_meas/1 -> Demux/1
  Demux/3 -> V->pu/1  "Vd Line"
  V->pu/1 -> [Vdc_line]
  Rectifier Controller/3(mode) -> [Mode_R]
  Rectifier Controller/2(Id_ref_lim) -> [Id_ref_lim_R]
  Rectifier Controller/1(alpha_ord (deg)) -> [alpha_ord_R], 12-pulse Firing Control/1(alpha_ord (deg))
  Demux/4 -> [Idc_pu]  "Idc"
  [VdL_R] -> Rectifier Controller/1(VdL (pu))
  Ground/1 -> Rectifier Controller/7(gamma_meas (deg)), Rectifier Controller/4(Vd_ref (pu)), Rectifier Controller/9(D_alpha (deg)), Rectifier Controller/8(gamma_ref (deg))
  Stop_R/1 -> Data Type Conversion/1
  Logical Operator3/1 -> Rectifier Protections/3(Deblocked)
  [VdL_R] -> Rectifier Protections/2(VdL (pu))
  Demux/1 -> 12-pulse Firing Control/2(Vabc (pu)), Rectifier Protections/1(Uabc (pu))  "Vabc"
  Data Type Conversion/1 -> Discrete Monostable/1, Discrete On/Off Delay/1
  Rectifier Protections/1(Forced_alpha) -> Logical Operator2/2
  Discrete On/Off Delay/1 -> 12-pulse Firing Control/3(Block), Rectifier Controller/5(Block), Logical Operator3/1
  Discrete Monostable/1 -> Logical Operator2/1
  Rectifier Protections/2(Low_ac_voltage) -> Data Type Conversion1/1
  Low_ac_inv/1 -> Rectifier Protections/4(Low_ac_volt_oth)

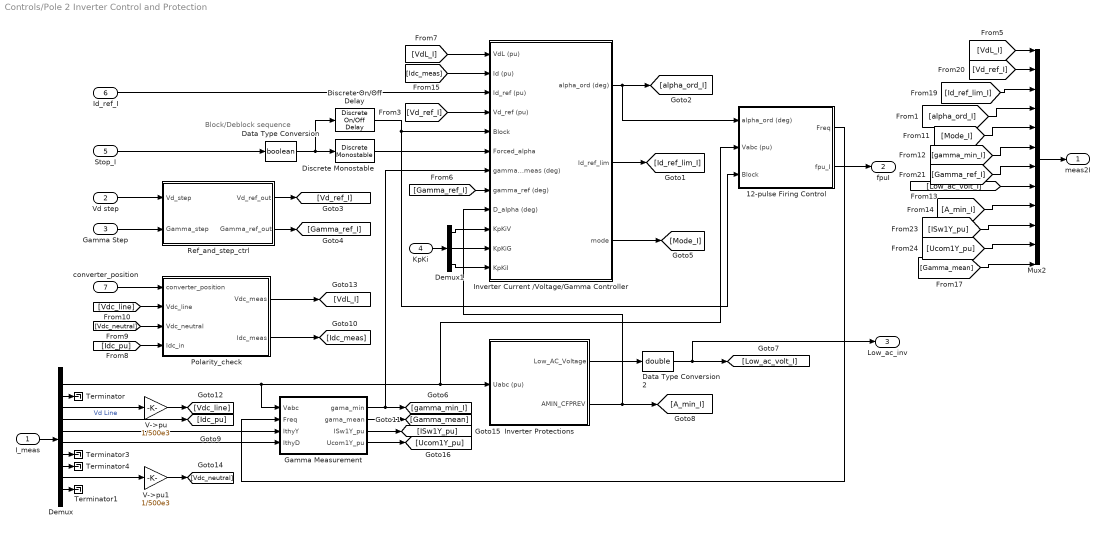
== system Controls/Pole 2 Inverter Control and Protection ==
  note: Block/Deblock sequence
  I_meas : Inport
  Vd step : Inport  Port=2
  Gamma Step : Inport  Port=3
  KpKi : Inport  Port=4
  Stop_I : Inport  Port=5
  Id_ref_I : Inport  Port=6
  converter_position : Inport  Port=7
  12-pulse Firing Control : Subsystem  mask(HVDC Discrete 12-pulse Firing Control){Pw=101.5, PLL_PF=[0,  50], PLL_G=[60, 1400], dt=Tctrl}
      mask prompts: Pw "{Pulse Generator}: Pulse Width (deg)"; PLL_PF "{PLL}: Initial [Phase (deg) Frequency (Hz)]"; PLL_G "{PLL}: Regulator gains [Kp (rad)  Ki (rad/s)]"; dt "Sample Time (s):"
      mask help:
      | This block contains a PLL and a 12-pulse generator to provide the firing pulses to the HVDC converter.
      | The firing control is of the equidistant type. It is based on a Phase Locked Loop (PLL) synchronized on positive-sequence of the fundamental voltage.
      mask init:
      | PLL_ph = PLL_PF(1); PLL_f0 = PLL_PF(2);
      | PLL_Kp = PLL_G(1); PLL_Ki = PLL_G(2);
      mask Help:
      | INPUTS:
      | alpha :  Desired firing angle of thyristors (deg).
      | Vabc  : 3 phase-to-ground voltages (pu)  on the primary winding of the YgYD converter transformer
      | Block  : Logical signal  (0-1). The pulses are not generated when the value is 1.
      | 
      | 
      | 
      | OUTPUTS:
      |  PulsesY :  6 pulses to be sent to the half converter connected to the Wye winding.
      |  PulsesD :  6 pulses to be sent to the half converter connected to the Delta winding.
  Data Type Conversion : DataTypeConversion  OutDataTypeStr=boolean
  Data Type Conversion2 : DataTypeConversion  OutDataTypeStr=double
  Demux : Demux  Outputs="[3 3 1 1 6 6 1  1 1 1]"
  Demux1 : Demux  Outputs=[2 2 2]
  Discrete Monostable : powerlib_extras/Discrete  Control Blocks/Discrete Monostable  EdgeDetect=Rising  t_mono=0.15  ic=1  Ts=Tctrl
  Discrete On/Off Delay : powerlib_extras/Discrete  Control Blocks/Discrete On//Off Delay  type_delay=On delay  delay=0.1  ic=1  Ts=Tctrl
  Gamma Measurement : Subsystem
  "Inverter Current /Voltage/Gamma Controller " : Subsystem  mask(Discrete HVDC Controller){Mode=Inverter (Current + Voltage + Gamma), XPILim=[166, 92], XLin=[160, 120], XKPI_I=[45, 4500, 90], Id_marg=0.1, XKPI_V=[35, 2250,  90], Vd_marg=0.05, XKPI_G=[1, 20,  90 ], G_marg=1, T_I=0.3e-3, XT_V=[15,  0.707], Xvdcol=[0.6, 0.18, 0.30, 0.1, 0.080], alpha_const=off, Xalpha_fix=[92, inf, -1000], dt=Tctrl}
      mask prompts: Mode "Control Mode :"; XPILim "{Alpha Limits}  [alpha max (deg), alpha min (deg) ]"; XLin "Kp Lin. Angle Limits (alpha or beta) : [Max  (deg), Min  (deg) ]"; XKPI_I "{Current Regulator}   [Kp (deg/pu) , Ki (deg/pu/s), AlphaInit (deg) ]"; Id_marg "Current Margin (pu) :"; XKPI_V "{Voltage Regulator}   [Kp (deg/pu) , Ki (deg/pu/s),  AlphaInit (deg) ]"; Vd_marg "Voltage Margin (pu):"; XKPI_G "{Gamma Regulator} [Kp, Ki (s), AlphaInit (deg)]"; G_marg "Gamma Margin (deg):"; T_I "{Id Meas. Filter H(s)=1/(1+Ts)} T(s):"; XT_V "{Vd Meas. Low-Pass 2nd Order Filter}  [fo,  Zeta ]"; Xvdcol "{VDCOL}  [ VdThresh.(pu),VdMin(pu),IdMin(pu),IdMinAbs(pu),Tup(s) ]"; alpha_const "Constant alpha mode"; Xalpha_fix "{Ct.  or Forced alpha)}  [Alpha (deg), + Rate limit, - Rate limit (deg/s)]"; dt "Sample Time (s):"
      mask help:
      | This block contains the regulators and functions to control the firing angle alpha of a HVDC rectifier or inverter.
      |  See the 'HVDC Transmission System' case study of the User's Manual for description of the block functionality.
      mask init: same as Controls/Pole 1 Inverter Control and Protection/Inverter Current /Voltage/Gamma Controller 
      mask TypeOptions Mode: Rectifier (Current) | Inverter (Current + Voltage + Gamma) | Inverter (Current + Voltage) | Inverter (Current + Gamma)
      mask Callback Mode:
      | mode=get_param(gcb,'Mode');
      | 
      | cb=get_param(gcb,'MaskVisibilities');
      | 
      | if strcmp(mode,'Rectifier (Current)')
      | 	cb{10}='on';
      |     cb{11} = 'off';
      | 
      | 	 cb{3}='off';
      | 	 cb{5}='off';cb{6}='off';cb{7}='off';cb{8}='off';cb{9}='off';
      |     set_param(gcb,'MaskVisibilities',cb);
      | elseif (strcmp(mode,'Inverter (Current + Voltage + Gamma)'))
      | 	 cb{3}='off';
      | 	 cb{5}='on';cb{6}='on';cb{7}='on';cb{8}='on';cb{9}='on';cb{11} = 'on';
      | 	 set_param(gcb,'MaskVisibilities',cb);
      | elseif (strcmp(mode,'Inverter (Current + Voltage)'))
      | 	 cb{3}='off';
      | 	 cb{5}='on';cb{6}='on';cb{7}='on';cb{8}='off';cb{9}='off'; cb{11} = 'on';
      |      set_param(gcb,'MaskVisibilities',cb);
      | else
      | 	 cb{3}='off';
      | 	 cb{5}='on';cb{6}='off';cb{7}='off';cb{8}='on';cb{9}='on'; cb{11} = 'on';
      | 	 set_param(gcb,'MaskVisibilities',cb);
      | end
  Inverter Protections : Subsystem  TreatAsAtomicUnit=on  mask(Protection LACVD a Radisson (cyc = 1 ms)){}
  Mux2 : Mux  Inputs=12
  Polarity_check : Subsystem
  Ref_and_step_ctrl : Subsystem
  Terminator{,1,3..4} (4 alike) : Terminator
  V->pu : Gain  Gain=1/500e3  SaturateOnIntegerOverflow=on  OutDataTypeStr=Inherit: Same as input  ParamDataTypeStr=Inherit: Same as input
  V->pu1 : Gain  Gain=1/500e3  SaturateOnIntegerOverflow=on  OutDataTypeStr=Inherit: Same as input  ParamDataTypeStr=Inherit: Same as input
  meas2I : Outport
  fpuI : Outport  Port=2
  Low_ac_inv : Outport  Port=3
  wires:
  V->pu1/1 -> [Vdc_neutral]
  Gamma Measurement/4(Ucom1Y_pu) -> [Ucom1Y_pu]
  Gamma Measurement/3(ISw1Y_pu) -> [ISw1Y_pu]
  Demux/1 -> 12-pulse Firing Control/2(Vabc (pu)), Inverter Protections/1(Uabc (pu)), Gamma Measurement/1(Vabc)
  [Idc_meas] -> "Inverter Current /Voltage/Gamma Controller "/2(Id (pu))
  Demux/9 -> V->pu1/1
  Demux/10 -> Terminator1/1
  Polarity_check/2(Idc_meas) -> [Idc_meas]
  [Vdc_neutral] -> Polarity_check/3(Vdc_neutral)
  [Vdc_line] -> Polarity_check/2(Vdc_line)
  converter_position/1 -> Polarity_check/1(converter_position)
  Polarity_check/1(Vdc_meas) -> [VdL_I]
  [Idc_pu] -> Polarity_check/4(Idc_in)
  Gamma Step/1 -> Ref_and_step_ctrl/2(Gamma_step)
  Ref_and_step_ctrl/2(Gamma_ref_out) -> [Gamma_ref_I]
  Vd step/1 -> Ref_and_step_ctrl/1(Vd_step)
  Ref_and_step_ctrl/1(Vd_ref_out) -> [Vd_ref_I]
  Demux1/1 -> "Inverter Current /Voltage/Gamma Controller "/10(KpKiV)
  Demux1/3 -> "Inverter Current /Voltage/Gamma Controller "/12(KpKiI)
  Demux1/2 -> "Inverter Current /Voltage/Gamma Controller "/11(KpKiG)
  KpKi/1 -> Demux1/1
  12-pulse Firing Control/2(fpu_I) -> fpuI/1
  12-pulse Firing Control/1(Freq) -> Gamma Measurement/2(Freq)
  Data Type Conversion2/1 -> Low_ac_inv/1, [Low_ac_volt_I]
  [Gamma_mean] -> Mux2/12
  [Ucom1Y_pu] -> Mux2/11
  [ISw1Y_pu] -> Mux2/10
  [A_min_I] -> Mux2/9
  [Low_ac_volt_I] -> Mux2/8
  [Gamma_ref_I] -> Mux2/7
  [gamma_min_I] -> Mux2/6
  [Mode_I] -> Mux2/5
  [alpha_ord_I] -> Mux2/4
  [Id_ref_lim_I] -> Mux2/3
  [Vd_ref_I] -> Mux2/2
  [VdL_I] -> Mux2/1
  Mux2/1 -> meas2I/1
  Demux/8 -> Terminator4/1
  Demux/7 -> Terminator3/1
  Demux/6 -> Gamma Measurement/4(IthyD)
  Demux/5 -> Gamma Measurement/3(IthyY)
  Demux/3 -> V->pu/1  "Vd Line"
  Demux/2 -> Terminator/1
  I_meas/1 -> Demux/1
  Discrete Monostable/1 -> "Inverter Current /Voltage/Gamma Controller "/6(Forced_alpha)
  [Vd_ref_I] -> "Inverter Current /Voltage/Gamma Controller "/4(Vd_ref (pu))
  Discrete On/Off Delay/1 -> 12-pulse Firing Control/3(Block), "Inverter Current /Voltage/Gamma Controller "/5(Block)
  Id_ref_I/1 -> "Inverter Current /Voltage/Gamma Controller "/3(Id_ref (pu))
  Demux/4 -> [Idc_pu]
  [VdL_I] -> "Inverter Current /Voltage/Gamma Controller "/1(VdL (pu))
  "Inverter Current /Voltage/Gamma Controller "/3(mode) -> [Mode_I]
  "Inverter Current /Voltage/Gamma Controller "/2(Id_ref_lim) -> [Id_ref_lim_I]
  "Inverter Current /Voltage/Gamma Controller "/1(alpha_ord (deg)) -> 12-pulse Firing Control/1(alpha_ord (deg)), [alpha_ord_I]
  Gamma Measurement/2(gama_mean) -> [Gamma_mean]
  Gamma Measurement/1(gama_min) -> [gamma_min_I], "Inverter Current /Voltage/Gamma Controller "/7(gamma_meas (deg))
  [Gamma_ref_I] -> "Inverter Current /Voltage/Gamma Controller "/8(gamma_ref (deg))
  V->pu/1 -> [Vdc_line]
  Inverter Protections/1(Low_AC_Voltage) -> Data Type Conversion2/1
  Inverter Protections/2(AMIN_CFPREV) -> "Inverter Current /Voltage/Gamma Controller "/9(D_alpha (deg)), [A_min_I]
  Stop_I/1 -> Data Type Conversion/1
  Data Type Conversion/1 -> Discrete Monostable/1, Discrete On/Off Delay/1

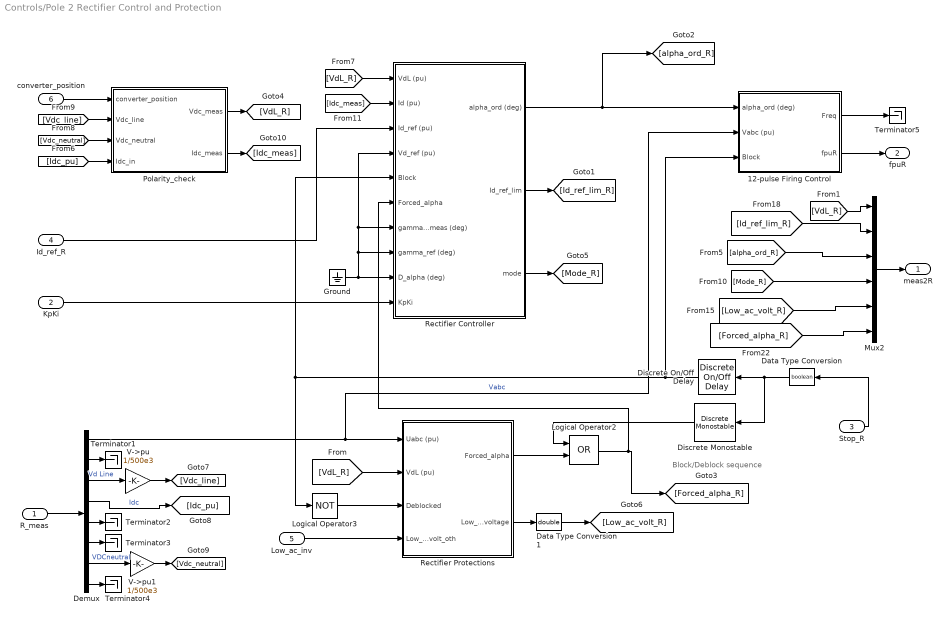
== system Controls/Pole 2 Rectifier Control and Protection ==
  note: Block/Deblock sequence
  R_meas : Inport
  KpKi : Inport  Port=2
  Stop_R : Inport  Port=3
  Id_ref_R : Inport  Port=4
  Low_ac_inv : Inport  Port=5
  converter_position : Inport  Port=6
  12-pulse Firing Control : Subsystem  mask(HVDC Discrete 12-pulse Firing Control){Pw=101.5, PLL_PF=[0,  60], PLL_G=[60, 1400], dt=Tctrl}
      mask prompts: Pw "{Pulse Generator}: Pulse Width (deg)"; PLL_PF "{PLL}: Initial [Phase (deg) Frequency (Hz)]"; PLL_G "{PLL}: Regulator gains [Kp (rad)  Ki (rad/s)]"; dt "Sample Time (s):"
      mask help:
      | This block contains a PLL and a 12-pulse generator to provide the firing pulses to the HVDC converter.
      | The firing control is of the equidistant type. It is based on a Phase Locked Loop (PLL) synchronized on positive-sequence of the fundamental voltage.
      mask init:
      | PLL_ph = PLL_PF(1); PLL_f0 = PLL_PF(2);
      | PLL_Kp = PLL_G(1); PLL_Ki = PLL_G(2);
      mask Help:
      | INPUTS:
      | alpha :  Desired firing angle of thyristors (deg).
      | Vabc  : 3 phase-to-ground voltages (pu)  on the primary winding of the YgYD converter transformer
      | Block  : Logical signal  (0-1). The pulses are not generated when the value is 1.
      | 
      | 
      | 
      | OUTPUTS:
      |  PulsesY :  6 pulses to be sent to the half converter connected to the Wye winding.
      |  PulsesD :  6 pulses to be sent to the half converter connected to the Delta winding.
  Data Type Conversion : DataTypeConversion  OutDataTypeStr=boolean
  Data Type Conversion1 : DataTypeConversion  OutDataTypeStr=double
  Demux : Demux  Outputs=[3 3 1 1 2 2 1 1]
  Discrete Monostable : powerlib_extras/Discrete  Control Blocks/Discrete Monostable  EdgeDetect=Rising  t_mono=0.15  ic=1  Ts=Tctrl
  Discrete On/Off Delay : powerlib_extras/Discrete  Control Blocks/Discrete On//Off Delay  type_delay=On delay  delay=0.1  ic=1  Ts=Tctrl
  Ground : Ground
  Logical Operator2 : Logic  Operator=OR  AllPortsSameDT=off
  Logical Operator3 : Logic  Operator=NOT
  Mux2 : Mux  Inputs=6
  Polarity_check : Subsystem
  Rectifier Controller : Subsystem  mask(Discrete HVDC Controller){Mode=Rectifier (Current), XPILim=[166, 5], XLin=[160, 120], XKPI_I=[45, 4500, 90], Id_marg=0.1, XKPI_V=[35, 2250,  90], Vd_marg=0.05, XKPI_G=[1, 20,  90 ], G_marg=1, T_I=0.3e-3, XT_V=[15,  0.707], Xvdcol=[0.6, 0.18, 0.30, 0.1, 0.080], alpha_const=off, Xalpha_fix=[166, inf, -inf], dt=Tctrl}
      mask prompts: Mode "Control Mode :"; XPILim "{Alpha Limits}  [alpha max (deg), alpha min (deg) ]"; XLin "Kp Lin. Angle Limits (alpha or beta) : [Max  (deg), Min  (deg) ]"; XKPI_I "{Current Regulator}   [Kp (deg/pu) , Ki (deg/pu/s), AlphaInit (deg) ]"; Id_marg "Current Margin (pu) :"; XKPI_V "{Voltage Regulator}   [Kp (deg/pu) , Ki (deg/pu/s),  AlphaInit (deg) ]"; Vd_marg "Voltage Margin (pu):"; XKPI_G "{Gamma Regulator} [Kp, Ki (s), AlphaInit (deg)]"; G_marg "Gamma Margin (deg):"; T_I "{Id Meas. Filter H(s)=1/(1+Ts)} T(s):"; XT_V "{Vd Meas. Low-Pass 2nd Order Filter}  [fo,  Zeta ]"; Xvdcol "{VDCOL}  [ VdThresh.(pu),VdMin(pu),IdMin(pu),IdMinAbs(pu),Tup(s) ]"; alpha_const "Constant alpha mode"; Xalpha_fix "{Ct.  or Forced alpha)}  [Alpha (deg), + Rate limit, - Rate limit (deg/s)]"; dt "Sample Time (s):"
      mask help:
      | This block contains the regulators and functions to control the firing angle alpha of a HVDC rectifier or inverter.
      |  See the 'HVDC Transmission System' case study of the User's Manual for description of the block functionality.
      mask init: same as Controls/Pole 1 Inverter Control and Protection/Inverter Current /Voltage/Gamma Controller 
      mask TypeOptions Mode: Rectifier (Current) | Inverter (Current + Voltage + Gamma) | Inverter (Current + Voltage) | Inverter (Current + Gamma)
      mask Callback Mode:
      | mode=get_param(gcb,'Mode');
      | 
      | cb=get_param(gcb,'MaskVisibilities');
      | 
      | if strcmp(mode,'Rectifier (Current)')
      | 	cb{10}='on';
      |     cb{11} = 'off';
      | 
      | 	 cb{3}='off';
      | 	 cb{5}='off';cb{6}='off';cb{7}='off';cb{8}='off';cb{9}='off';
      |     set_param(gcb,'MaskVisibilities',cb);
      | elseif (strcmp(mode,'Inverter (Current + Voltage + Gamma)'))
      | 	 cb{3}='off';
      | 	 cb{5}='on';cb{6}='on';cb{7}='on';cb{8}='on';cb{9}='on';cb{11} = 'on';
      | 	 set_param(gcb,'MaskVisibilities',cb);
      | elseif (strcmp(mode,'Inverter (Current + Voltage)'))
      | 	 cb{3}='off';
      | 	 cb{5}='on';cb{6}='on';cb{7}='on';cb{8}='off';cb{9}='off'; cb{11} = 'on';
      |      set_param(gcb,'MaskVisibilities',cb);
      | else
      | 	 cb{3}='off';
      | 	 cb{5}='on';cb{6}='off';cb{7}='off';cb{8}='on';cb{9}='on'; cb{11} = 'on';
      | 	 set_param(gcb,'MaskVisibilities',cb);
      | end
  Rectifier Protections : Subsystem  TreatAsAtomicUnit=on  mask(Protection LACVD a Radisson (cyc = 1 ms)){}
  Terminator{1..5} (5 alike) : Terminator
  V->pu : Gain  Gain=1/500e3  SaturateOnIntegerOverflow=on  OutDataTypeStr=Inherit: Same as input  ParamDataTypeStr=Inherit: Same as input
  V->pu1 : Gain  Gain=1/500e3  SaturateOnIntegerOverflow=on  OutDataTypeStr=Inherit: Same as input  ParamDataTypeStr=Inherit: Same as input
  meas2R : Outport
  fpuR : Outport  Port=2
  wires:
  Logical Operator2/1 -> [Forced_alpha_R], Rectifier Controller/6(Forced_alpha)
  V->pu1/1 -> [Vdc_neutral]
  Id_ref_R/1 -> Rectifier Controller/3(Id_ref (pu))
  [Idc_meas] -> Rectifier Controller/2(Id (pu))
  Polarity_check/2(Idc_meas) -> [Idc_meas]
  [Vdc_neutral] -> Polarity_check/3(Vdc_neutral)
  [Vdc_line] -> Polarity_check/2(Vdc_line)
  converter_position/1 -> Polarity_check/1(converter_position)
  Polarity_check/1(Vdc_meas) -> [VdL_R]
  [Idc_pu] -> Polarity_check/4(Idc_in)
  Demux/7 -> V->pu1/1  "VDCneutral"
  Demux/8 -> Terminator4/1
  KpKi/1 -> Rectifier Controller/10(KpKi)
  12-pulse Firing Control/2(fpuR) -> fpuR/1
  12-pulse Firing Control/1(Freq) -> Terminator5/1
  Data Type Conversion1/1 -> [Low_ac_volt_R]
  Mux2/1 -> meas2R/1
  [Forced_alpha_R] -> Mux2/6
  [Low_ac_volt_R] -> Mux2/5
  [Mode_R] -> Mux2/4
  [alpha_ord_R] -> Mux2/3
  [Id_ref_lim_R] -> Mux2/2
  [VdL_R] -> Mux2/1
  Demux/6 -> Terminator3/1
  Demux/5 -> Terminator2/1
  Demux/2 -> Terminator1/1
  R_meas/1 -> Demux/1
  Demux/3 -> V->pu/1  "Vd Line"
  V->pu/1 -> [Vdc_line]
  Rectifier Controller/3(mode) -> [Mode_R]
  Rectifier Controller/2(Id_ref_lim) -> [Id_ref_lim_R]
  Rectifier Controller/1(alpha_ord (deg)) -> [alpha_ord_R], 12-pulse Firing Control/1(alpha_ord (deg))
  Demux/4 -> [Idc_pu]  "Idc"
  [VdL_R] -> Rectifier Controller/1(VdL (pu))
  Ground/1 -> Rectifier Controller/9(D_alpha (deg)), Rectifier Controller/8(gamma_ref (deg)), Rectifier Controller/7(gamma_meas (deg)), Rectifier Controller/4(Vd_ref (pu))
  Stop_R/1 -> Data Type Conversion/1
  Logical Operator3/1 -> Rectifier Protections/3(Deblocked)
  [VdL_R] -> Rectifier Protections/2(VdL (pu))
  Demux/1 -> 12-pulse Firing Control/2(Vabc (pu)), Rectifier Protections/1(Uabc (pu))  "Vabc"
  Data Type Conversion/1 -> Discrete Monostable/1, Discrete On/Off Delay/1
  Rectifier Protections/1(Forced_alpha) -> Logical Operator2/2
  Discrete On/Off Delay/1 -> 12-pulse Firing Control/3(Block), Rectifier Controller/5(Block), Logical Operator3/1
  Discrete Monostable/1 -> Logical Operator2/1
  Rectifier Protections/2(Low_ac_voltage) -> Data Type Conversion1/1
  Low_ac_inv/1 -> Rectifier Protections/4(Low_ac_volt_oth)
